simulink model "modelo_linear_0"  (R2013a)
settings: Solver=ode45  StartTime=0.0  StopTime=0.8  RelTol=1e-3
values from neighbouring files (symbols this model uses):
  gb = 0.3e-3    (= 0.0003)    [parametriza.m]    (also in parametrizaMancal.m)
  Kb = 58    [parametriza.m]    (also in parametrizaMancal.m = E*Hb*Ab/Lb)
  Kp = 625    [parametriza.m]
  L2 = 7.807e-05    [parametriza.m]
  m = 0.375    [parametriza.m]    (also in parametrizaMancal.m)
  R = 6.3    [parametriza.m]    (also in parametrizaMancal.m = 6)
libraries: simulink x2
settings Model: Creator=corsi  LastModifiedBy=rafa
settings OptimizationCC: ExpressionDepthLimit=2147483647

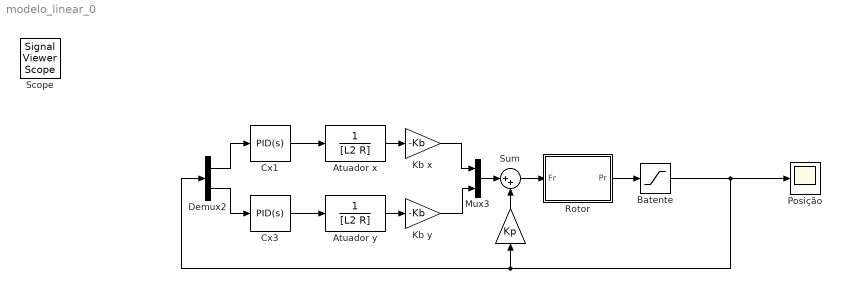
== system modelo_linear_0 ==
  " " : Gain  Gain=Kp
  Atuador x : TransferFcn  Denominator=[L2 R]
  "Atuador y " : TransferFcn  Denominator=[L2 R]
  Batente : Saturate  UpperLimit=gb  LowerLimit=-gb
  Cx1 : simulink/Continuous/PID Controller  Controller=PID  TimeDomain=Continuous-time  SampleTime=1  IntegratorMethod=Forward Euler  FilterMethod=Forward Euler  Form=Ideal  P=1926.82458055705  I=5.89623132861836  D=0.0171863241690584  N=1616.33345877961  InitialConditionSource=internal  InitialConditionForIntegrator=0  InitialConditionForFilter=0  ExternalReset=none  LimitOutput=off  UpperSaturationLimit=inf  LowerSaturationLimit=-inf  LinearizeAsGain=on  AntiWindupMode=none  Kb=1  TrackingMode=off  Kt=1  PParamMin=[]  PParamMax=[]  IParamMin=[]  IParamMax=[]  DParamMin=[]  DParamMax=[]  NParamMin=[]  NParamMax=[]  KbParamMin=[]  KbParamMax=[]  KtParamMin=[]  KtParamMax=[]  POutMin=[]  POutMax=[]  IOutMin=[]  IOutMax=[]  DOutMin=[]  DOutMax=[]  NOutMin=[]  NOutMax=[]  KbOutMin=[]  KbOutMax=[]  KtOutMin=[]  KtOutMax=[]  IntegratorOutMin=[]  IntegratorOutMax=[]  FilterOutMin=[]  FilterOutMax=[]  SumOutMin=[]  SumOutMax=[]  SumI1OutMin=[]  SumI1OutMax=[]  SumI2OutMin=[]  SumI2OutMax=[]  SumI3OutMin=[]  SumI3OutMax=[]  SumDOutMin=[]  SumDOutMax=[]  SaturationOutMin=[]  SaturationOutMax=[]  IntegratorContinuousStateAttributes=''  IntegratorStateMustResolveToSignalObject=off  IntegratorRTWStateStorageClass=Auto  FilterContinuousStateAttributes=''  FilterStateMustResolveToSignalObject=off  FilterRTWStateStorageClass=Auto
  Cx3 : simulink/Continuous/PID Controller  Controller=PID  TimeDomain=Continuous-time  SampleTime=1  IntegratorMethod=Forward Euler  FilterMethod=Forward Euler  Form=Ideal  P=1926.82458055705  I=5.89623132861836  D=0.0171863241690584  N=1616.33345877961  InitialConditionSource=internal  InitialConditionForIntegrator=0  InitialConditionForFilter=0  ExternalReset=none  LimitOutput=off  UpperSaturationLimit=inf  LowerSaturationLimit=-inf  LinearizeAsGain=on  AntiWindupMode=none  Kb=1  TrackingMode=off  Kt=1  PParamMin=[]  PParamMax=[]  IParamMin=[]  IParamMax=[]  DParamMin=[]  DParamMax=[]  NParamMin=[]  NParamMax=[]  KbParamMin=[]  KbParamMax=[]  KtParamMin=[]  KtParamMax=[]  POutMin=[]  POutMax=[]  IOutMin=[]  IOutMax=[]  DOutMin=[]  DOutMax=[]  NOutMin=[]  NOutMax=[]  KbOutMin=[]  KbOutMax=[]  KtOutMin=[]  KtOutMax=[]  IntegratorOutMin=[]  IntegratorOutMax=[]  FilterOutMin=[]  FilterOutMax=[]  SumOutMin=[]  SumOutMax=[]  SumI1OutMin=[]  SumI1OutMax=[]  SumI2OutMin=[]  SumI2OutMax=[]  SumI3OutMin=[]  SumI3OutMax=[]  SumDOutMin=[]  SumDOutMax=[]  SaturationOutMin=[]  SaturationOutMax=[]  IntegratorContinuousStateAttributes=''  IntegratorStateMustResolveToSignalObject=off  IntegratorRTWStateStorageClass=Auto  FilterContinuousStateAttributes=''  FilterStateMustResolveToSignalObject=off  FilterRTWStateStorageClass=Auto
  Demux2 : Demux  Outputs=2
  Kb x : Gain  Gain=-Kb
  Kb y : Gain  Gain=-Kb
  Mux3 : Mux  Inputs=2
  Posição : Scope
      settings: YMin=-3e-07  YMax=2e-06
  Rotor : Subsystem
  Sum : Sum  Inputs=|++
  Scope : SignalViewerScope  IOType=viewer  RefreshTime=0.035000
  wires:
  Atuador x/1 -> Kb x/1
  Rotor/1(Pr) -> Batente/1
  "Atuador y "/1 -> Kb y/1
  Demux2/1 -> Cx1/1
  Demux2/2 -> Cx3/1
  Kb y/1 -> Mux3/2
  Kb x/1 -> Mux3/1
  Mux3/1 -> Sum/1
  Sum/1 -> Rotor/1(Fr)
  " "/1 -> Sum/2
  Batente/1 -> Posição/1, Demux2/1, " "/1
  Cx3/1 -> "Atuador y "/1
  Cx1/1 -> Atuador x/1

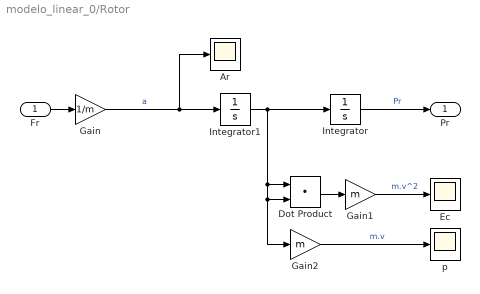
== system modelo_linear_0/Rotor ==
  Fr : Inport
  Ar : Scope
      settings: TimeRange=1  YMin=-200000  YMax=200000  SaveName=ScopeData9
  Dot Product : DotProduct  InputSameDT=on  OutDataTypeStr=Inherit: Inherit via internal rule
  Ec : Scope
      settings: TimeRange=0.25  YMin=0  YMax=0.09  SaveName=ScopeData16
  Gain : Gain  Gain=1/m
  Gain1 : Gain  Gain=m
  Gain2 : Gain  Gain=m
  Integrator : Integrator  InitialCondition=[.001 .002]*1e-3  UpperSaturationLimit=Inf  LowerSaturationLimit=-Inf
  Integrator1 : Integrator
  p : Scope
      settings: TimeRange=1  YMin=-200000  YMax=200000  SaveName=ScopeData17
  Pr : Outport
  wires:
  Fr/1 -> Gain/1
  Integrator/1 -> Pr/1  "Pr"
  Gain/1 -> Ar/1, Integrator1/1  "a"
  Dot Product/1 -> Gain1/1
  Integrator1/1 -> Dot Product/1, Gain2/1, Dot Product/2, Integrator/1
  Gain2/1 -> p/1  "m.v"
  Gain1/1 -> Ec/1  "m.v^2"
